simulink model "untitled2"  (R2022b)
settings: Solver=ode45  StartTime=0.0  StopTime=10.0  RelTol=1e-3  EnableMultiTasking=on
settings Model: Creator=autologin  LastModifiedBy=AMD
settings SolverCC: AlgebraicLoopSolver=TrustRegion
settings DataIOCC: LimitDataPoints=on  SaveFormat=Array  SignalLoggingSaveFormat=ModelDataLogs  ReturnWorkspaceOutputs=off
settings OptimizationCC: ExpressionDepthLimit=2147483647  LifeSpan=inf
settings DebuggingCC: UnderspecifiedInitializationDetection=Classic  MergeDetectMultiDrivingBlocksExec=none  SolverPrmCheckMsg=warning  FcnCallInpInsideContextMsg=warning  UnconnectedInputMsg=warning  UnconnectedOutputMsg=warning  UnconnectedLineMsg=warning  StateNameClashWarn=warning  SFUnexpectedBacktrackingDiag=warning  SFNoUnconditionalDefaultTransitionDiag=warning  SFExecutionAtInitializationDiag=none  SFMachineParentedDataDiag=warning  ArithmeticOperatorsInVariantConditions=warning
settings HardwareCC: ProdBitPerPointer=32  ProdBitPerSizeT=32  ProdBitPerPtrDiffT=32  ProdLargestAtomicFloat=None  ProdIntDivRoundTo=Undefined  ProdEndianess=Unspecified  ProdWordSize=32  ProdHWDeviceType=32-bit Generic
settings ModelReferenceCC: PropagateSignalLabelsOutOfModel=off
settings SFSimCC: SimUseLocalCustomCode=off  CustomCodeUndefinedFunction=UseInterfaceOnly
settings RTWCC: RTWUseLocalCustomCode=off
settings CodeAppCC: StateflowObjectComments=on
settings GRTTargetCC: TargetLangStandard=C89/C90 (ANSI)  CombineOutputUpdateFcns=off  GRTInterface=on
settings ConfigComp: CovMetricSettings=dw  CovSaveCumulativeToWorkspaceVar=on  CovSaveSingleToWorkspaceVar=on  CovExternalEMLEnable=off

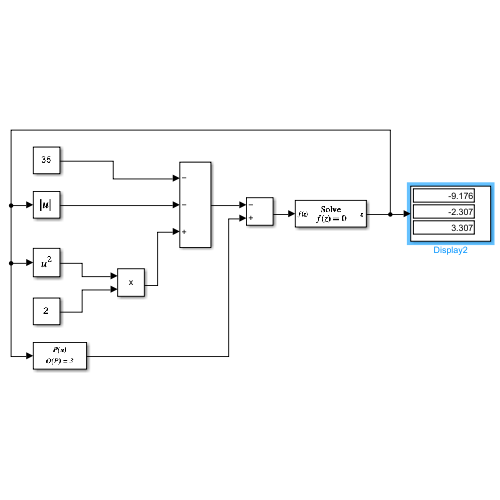
[thumbnail: Simulink's stored preview of the top-level diagram]
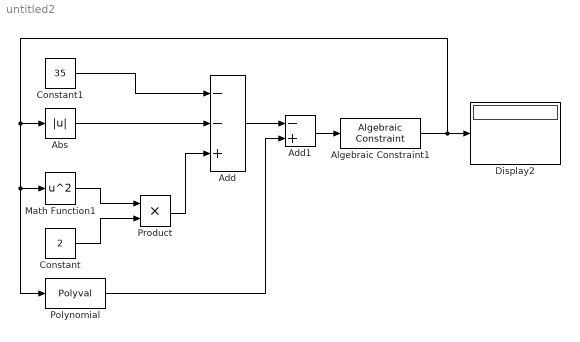
== system untitled2 ==
  Abs : Abs  SaturateOnIntegerOverflow=off
  Add : Sum  Inputs=--+
  Add1 : Sum  Inputs=-+
  Algebraic Constraint1 : AlgebraicConstraint  InitialGuess=[-9, -3, 3]
  Constant : Constant  Value=2
  Constant1 : Constant  Value=35
  Display2 : Display
  Math Function1 : Math  Operator=square  SignedPower=on
  Polynomial : Polyval  Coefs=[-0.6, -3, 10, 5]
  Product : Product  RndMeth=Zero
  wires:
  Math Function1/1 -> Product/1
  Constant/1 -> Product/2
  Product/1 -> Add/3
  Constant1/1 -> Add/1
  Abs/1 -> Add/2
  Algebraic Constraint1/1 -> Polynomial/1, Math Function1/1, Abs/1, Display2/1
  Add/1 -> Add1/1
  Polynomial/1 -> Add1/2
  Add1/1 -> Algebraic Constraint1/1
